simulink model "scopeInterface"  (R2023b)
settings: Solver=FixedStepAuto  StartTime=0.0  StopTime=30  FixedStep=0.01  RelTol=1e-3
undefined symbols (not defined in the file or in its folder): param
settings Model: PacingRate=1.530000  Creator=Scott.Dahlke  LastModifiedBy=Connor Emmons
settings SolverCC: AlgebraicLoopSolver=TrustRegion
settings DebuggingCC: UnconnectedInputMsg=warning  UnconnectedOutputMsg=warning  UnconnectedLineMsg=warning
settings ModelReferenceCC: EnableRefExpFcnMdlSchedulingChecks=on
settings SFSimCC: CustomCodeUndefinedFunction=UseInterfaceOnly
settings RTWCC: DLArmComputeVersion=19.05

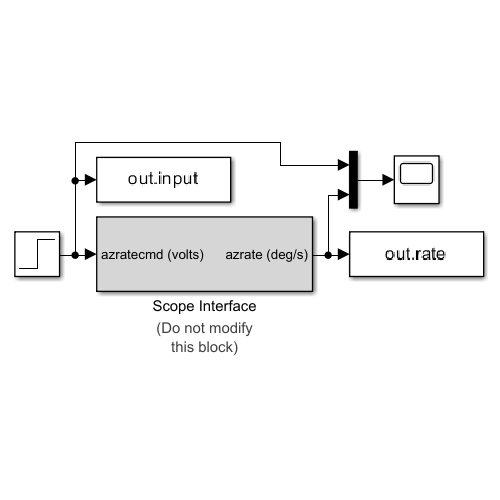
[thumbnail: Simulink's stored preview of the top-level diagram]
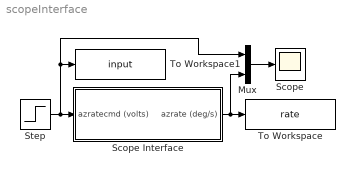
== system scopeInterface ==
  Mux : Mux  Inputs=2
  Scope : Scope
  Scope Interface : Subsystem
      settings: AttributesFormatString=|
      | (Do not modify
      | this block)
  Step : Step  SampleTime=0
  To Workspace : ToWorkspace  VariableName=rate  SampleTime=-1
  To Workspace1 : ToWorkspace  VariableName=input  SampleTime=-1
  wires:
  Step/1 -> Mux/1, To Workspace1/1, Scope Interface/1(azratecmd (volts))
  Scope Interface/1(azrate (deg/s)) -> Mux/2, To Workspace/1
  Mux/1 -> Scope/1

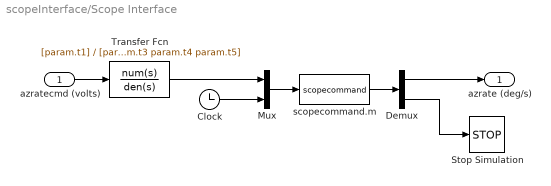
== system scopeInterface/Scope Interface ==
  azratecmd (volts) : Inport
  Clock : Clock
  Demux : Demux  Outputs=2
  Mux : Mux  Inputs=2
  Stop Simulation : Stop
  Transfer Fcn : TransferFcn  Numerator=[param.t1]  Denominator=[param.t3 param.t4 param.t5]
  scopecommand.m : MATLABFcn  MATLABFcn=scopecommand  OutputDimensions=2
  azrate (deg/s) : Outport
  wires:
  azratecmd (volts)/1 -> Transfer Fcn/1
  Mux/1 -> scopecommand.m/1
  Demux/2 -> Stop Simulation/1
  Demux/1 -> azrate (deg/s)/1
  scopecommand.m/1 -> Demux/1
  Transfer Fcn/1 -> Mux/1
  Clock/1 -> Mux/2
